simulink model "MATLAB Simulink Model"  (R2020b)
settings: Solver=ode4  StartTime=0.0  StopTime=1  RelTol=1e-3
InitFcn:
  | clear;
  | clc;
  | 
  | %Motor Parameters
  | r1 = 1.405;
  | l1  = 0.005839;
  | r2 = 1.395;
  | l2 = 0.005839;
  | Lm = 0.1722;
  | 
  | %Motor Rated Values
  | Vrat = 400;
  | frat = 50;
  | 
  | x1 = 2*pi*frat*l1;
  | x2 = 2*pi*frat*l2;
  | Xm = 2*pi*frat*Lm;
  | Prat = 4*1000;
  | Nrat = 1430;
  | Ns = 120*frat/4;
  | nrat = Nrat*2*pi/60;
  | ns = Ns*2*pi/60;
  | srat = (Ns-Nrat)/Ns;
  | 
  | E1 = Vrat/sqrt(3); %phase voltage
  | IL = E1/( (r1 + (1i*x1) ) + ( ( (1i*x2) +(r2/srat) )*1i*Xm / ( (1i*Xm) + (1i*x2) + (r2/srat) ) ) );
  | E2 = E1 - (IL*(r1 + (1i*x1) ) );
  | Trat = (3/(ns))*srat*abs(E2)*abs(E2)*r2/((r2*r2) + (srat*srat*x2*x2));
  | %Trat = Prat/nrat;
  | 
  | %System Variables
  | Tsys = (1e-6);
  | Ts = (100e-6);
  | freq = 50;
  | 
  | m=1*freq/50;
  | %m = 1 * (freq/50);
  | Vbus = (400*sqrt(2)*2/sqrt(3)) / (1.15);
  | 
  | Vref = (Vbus*sqrt(3)/2) * m;
  | delay = Ts/Tsys;
  | 
  | % Motor Starting Parameters
  | inc_time = 0.1;
  | 
  | %Motor Loading time
  | load_time = 0.5;
  | 
  | %No. of Hybrid Zones
  | numzones = 3;
  | 
  | %Load ML model Weights
  | 
  | W1R_s1 = readmatrix('Regression Weights\W1_subnet1_tmp_odd_90.xlsx');
  | b1R_s1 = readmatrix('Regression Weights\b1_subnet1_tmp_odd_90.xlsx');
  | W1R_s2 = readmatrix('Regression Weights\W1_subnet2_tmp_odd_90.xlsx');
  | b1R_s2 = readmatrix('Regression Weights\b1_subnet2_tmp_odd_90.xlsx');
  | 
  | W2R = readmatrix('Regression Weights\W2_subnet_tmp_odd_90.xlsx');
  | b2R = readmatrix('Regression Weights\b2_subnet_tmp_odd_90.xlsx');
  | ... (+9 lines)
libraries: powerlib x72, simulink x55, powerlib_meascontrol x15, dspstat3 x11, dspsigops x1
(part 3 of 5)

== system MATLAB Simulink Model/Space Vector PWM based VSI 1/Gating Pulse Generator/Gate Pulse Generator for 2721 Sequence ==
  "S1, S3, S5, sector" : Inport
  AND{,1..5} (6 alike) : Logic  IconShape=distinctive  AllPortsSameDT=off  OutDataTypeStr=boolean
  Constant : Constant  Value=2
  Data Type Conversion : DataTypeConversion
  Demux : Demux
  For Even Sector : Subsystem
  For Odd Sector : Subsystem
  Mod : Math  Operator=mod  SaturateOnIntegerOverflow=on
  Mux : Mux  Inputs=3
  NOT : Logic  Operator=NOT  IconShape=distinctive  AllPortsSameDT=off  OutDataTypeStr=boolean
  OR : Logic  Operator=OR  IconShape=distinctive  AllPortsSameDT=off  OutDataTypeStr=boolean
  OR1 : Logic  Operator=OR  IconShape=distinctive  AllPortsSameDT=off  OutDataTypeStr=boolean
  OR2 : Logic  Operator=OR  IconShape=distinctive  AllPortsSameDT=off  OutDataTypeStr=boolean
  Scope1 : Scope  NumInputPorts=4
  Gate 1 Pulse : Outport
  Gate 3 Pulse : Outport  Port=2
  Gate 5 Pulse : Outport  Port=3
  wires:
  For Even Sector/1(Gate 1 Pulse) -> AND/1
  NOT/1 -> AND2/2, AND1/2, AND/2
  Constant/1 -> Mod/2
  Mux/1 -> For Odd Sector/1("S1, S3, S1"), For Even Sector/1("S1, S3, S5")
  Demux/1 -> Mux/1
  Demux/4 -> Mod/1, Scope1/4
  AND3/1 -> OR/1
  "S1, S3, S5, sector"/1 -> Demux/1
  AND2/1 -> OR2/2
  Data Type Conversion/1 -> NOT/1, AND5/2, AND4/2, AND3/2
  Mod/1 -> Data Type Conversion/1
  AND/1 -> OR/2
  AND1/1 -> OR1/2
  For Odd Sector/2(Gate 3 Pulse) -> AND4/1
  Demux/2 -> Mux/2
  AND5/1 -> OR2/1
  OR/1 -> Gate 1 Pulse/1, Scope1/1
  AND4/1 -> OR1/1
  Demux/3 -> Mux/3
  OR1/1 -> Gate 3 Pulse/1, Scope1/2
  For Even Sector/2(Gate 3 Pulse) -> AND1/1
  OR2/1 -> Gate 5 Pulse/1, Scope1/3
  For Even Sector/3(Gate 5 Pulse) -> AND2/1
  For Odd Sector/1(Gate 1 Pulse) -> AND3/1
  For Odd Sector/3(Gate 5 Pulse) -> AND5/1

== system MATLAB Simulink Model/Space Vector PWM based VSI 1/Gating Pulse Generator/Gate Pulse Generator for 7212 Sequence ==
  "S1, S3, S5, sector" : Inport
  AND{,1..5} (6 alike) : Logic  IconShape=distinctive  AllPortsSameDT=off  OutDataTypeStr=boolean
  Constant : Constant  Value=2
  Data Type Conversion : DataTypeConversion
  Demux : Demux
  For Even Sector : Subsystem
  For Odd Sector : Subsystem
  Mod : Math  Operator=mod  SaturateOnIntegerOverflow=on
  Mux : Mux  Inputs=3
  NOT : Logic  Operator=NOT  IconShape=distinctive  AllPortsSameDT=off  OutDataTypeStr=boolean
  OR : Logic  Operator=OR  IconShape=distinctive  AllPortsSameDT=off  OutDataTypeStr=boolean
  OR1 : Logic  Operator=OR  IconShape=distinctive  AllPortsSameDT=off  OutDataTypeStr=boolean
  OR2 : Logic  Operator=OR  IconShape=distinctive  AllPortsSameDT=off  OutDataTypeStr=boolean
  Scope1 : Scope  NumInputPorts=4
  Gate 1 Pulse : Outport
  Gate 3 Pulse : Outport  Port=2
  Gate 5 Pulse : Outport  Port=3
  wires:
  AND3/1 -> OR/1
  "S1, S3, S5, sector"/1 -> Demux/1
  For Odd Sector/2(Gate 3 Pulse) -> AND4/1
  NOT/1 -> AND2/2, AND1/2, AND/2
  Constant/1 -> Mod/2
  Mux/1 -> For Odd Sector/1("S1, S3, S5"), For Even Sector/1("S1, S3, S1")
  Demux/1 -> Mux/1
  AND2/1 -> OR2/2
  Data Type Conversion/1 -> NOT/1, AND5/2, AND4/2, AND3/2
  Demux/4 -> Mod/1, Scope1/4
  Mod/1 -> Data Type Conversion/1
  AND/1 -> OR/2
  AND1/1 -> OR1/2
  Demux/2 -> Mux/2
  AND5/1 -> OR2/1
  OR/1 -> Gate 1 Pulse/1, Scope1/1
  AND4/1 -> OR1/1
  For Even Sector/1(Gate 1 Pulse) -> AND/1
  Demux/3 -> Mux/3
  OR1/1 -> Gate 3 Pulse/1, Scope1/2
  OR2/1 -> Gate 5 Pulse/1, Scope1/3
  For Even Sector/2(Gate 3 Pulse) -> AND1/1
  For Even Sector/3(Gate 5 Pulse) -> AND2/1
  For Odd Sector/1(Gate 1 Pulse) -> AND3/1
  For Odd Sector/3(Gate 5 Pulse) -> AND5/1

== system MATLAB Simulink Model/Space Vector PWM based VSI 1/Switching Times and Sector/Angle Calculation1 ==
  freq : Inport
  Delay : Delay  DelayLength=1  InitialCondition=0  UseCircularBuffer=on
  Gain1 : Gain  Gain=Tsys
  MATLAB Function : MATLAB Function  TreatAsAtomicUnit=on
  Scope : Scope
  Zero-Order Hold : ZeroOrderHold  SampleTime=Ts
  w : Gain  Gain=2*pi
  wt : Goto  Commented=on  GotoTag=wt  TagVisibility=global
  Angle : Outport
  wires:
  w/1 -> Gain1/1
  MATLAB Function/1(wnew) -> wt/1, Zero-Order Hold/1, Delay/1
  Delay/1 -> MATLAB Function/1(wold)
  Zero-Order Hold/1 -> Angle/1
  Gain1/1 -> MATLAB Function/2(wTs)
  freq/1 -> Scope/1, w/1

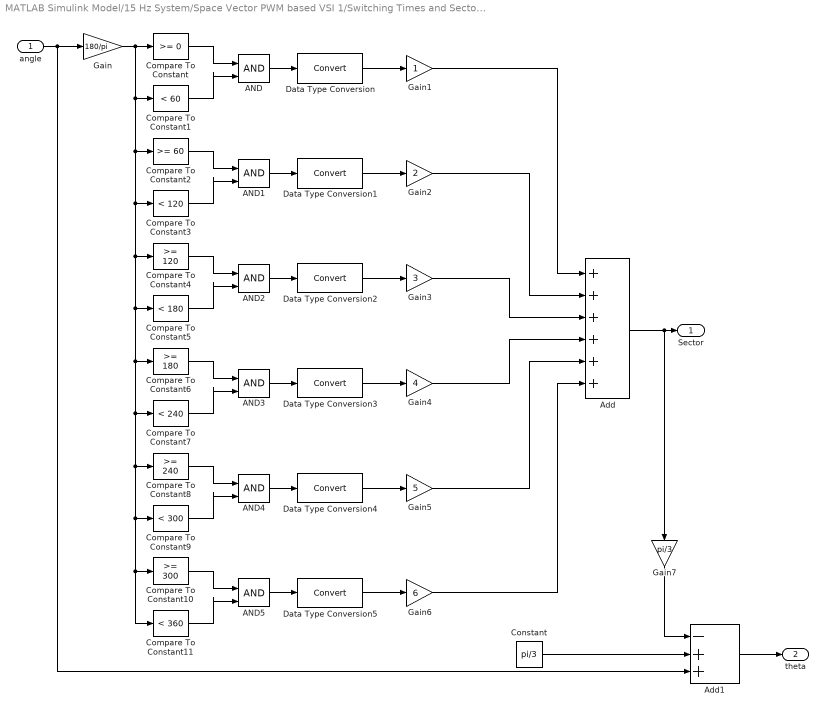
== system MATLAB Simulink Model/15 Hz System/Space Vector PWM based VSI 1/Switching Times and Sector/Angle to Sector and Theta ==
  angle : Inport
  AND{,1..5} (6 alike) : Logic  IconShape=distinctive  AllPortsSameDT=off  OutDataTypeStr=boolean
  Add : Sum  Inputs=++++++
  Add1 : Sum  Inputs=-++
  Compare To Constant : simulink/Logic and Bit Operations/Compare To Constant  relop=>=  const=0  OutDataTypeStr=boolean
  Compare To Constant1 : simulink/Logic and Bit Operations/Compare To Constant  relop=<  const=60  OutDataTypeStr=boolean
  Compare To Constant10 : simulink/Logic and Bit Operations/Compare To Constant  relop=>=  const=300  OutDataTypeStr=boolean
  Compare To Constant11 : simulink/Logic and Bit Operations/Compare To Constant  relop=<  const=360  OutDataTypeStr=boolean
  Compare To Constant2 : simulink/Logic and Bit Operations/Compare To Constant  relop=>=  const=60  OutDataTypeStr=boolean
  Compare To Constant3 : simulink/Logic and Bit Operations/Compare To Constant  relop=<  const=120  OutDataTypeStr=boolean
  Compare To Constant4 : simulink/Logic and Bit Operations/Compare To Constant  relop=>=  const=120  OutDataTypeStr=boolean
  Compare To Constant5 : simulink/Logic and Bit Operations/Compare To Constant  relop=<  const=180  OutDataTypeStr=boolean
  Compare To Constant6 : simulink/Logic and Bit Operations/Compare To Constant  relop=>=  const=180  OutDataTypeStr=boolean
  Compare To Constant7 : simulink/Logic and Bit Operations/Compare To Constant  relop=<  const=240  OutDataTypeStr=boolean
  Compare To Constant8 : simulink/Logic and Bit Operations/Compare To Constant  relop=>=  const=240  OutDataTypeStr=boolean
  Compare To Constant9 : simulink/Logic and Bit Operations/Compare To Constant  relop=<  const=300  OutDataTypeStr=boolean
  Constant : Constant  Value=pi/3
  Data Type Conversion{,1..5} (6 alike) : DataTypeConversion
  Gain : Gain  Gain=180/pi
  Gain1 : Gain
  Gain2 : Gain  Gain=2
  Gain3 : Gain  Gain=3
  Gain4 : Gain  Gain=4
  Gain5 : Gain  Gain=5
  Gain6 : Gain  Gain=6
  Gain7 : Gain  Gain=pi/3
  Sector : Outport
  theta : Outport  Port=2
  wires:
  Add/1 -> Gain7/1, Sector/1
  Gain6/1 -> Add/6
  Gain5/1 -> Add/5
  Gain2/1 -> Add/2
  Gain1/1 -> Add/1
  Gain3/1 -> Add/3
  Gain4/1 -> Add/4
  AND5/1 -> Data Type Conversion5/1
  Data Type Conversion5/1 -> Gain6/1
  Compare To Constant11/1 -> AND5/2
  Compare To Constant10/1 -> AND5/1
  AND4/1 -> Data Type Conversion4/1
  Data Type Conversion4/1 -> Gain5/1
  Compare To Constant9/1 -> AND4/2
  Compare To Constant8/1 -> AND4/1
  AND3/1 -> Data Type Conversion3/1
  Data Type Conversion3/1 -> Gain4/1
  Compare To Constant7/1 -> AND3/2
  Compare To Constant6/1 -> AND3/1
  AND2/1 -> Data Type Conversion2/1
  Data Type Conversion2/1 -> Gain3/1
  Compare To Constant5/1 -> AND2/2
  Compare To Constant4/1 -> AND2/1
  AND1/1 -> Data Type Conversion1/1
  Data Type Conversion1/1 -> Gain2/1
  Compare To Constant3/1 -> AND1/2
  Compare To Constant2/1 -> AND1/1
  Data Type Conversion/1 -> Gain1/1
  AND/1 -> Data Type Conversion/1
  Compare To Constant1/1 -> AND/2
  Compare To Constant/1 -> AND/1
  Gain/1 -> Compare To Constant1/1, Compare To Constant2/1, Compare To Constant3/1, Compare To Constant4/1, Compare To Constant5/1, Compare To Constant6/1, Compare To Constant7/1, Compare To Constant8/1, Compare To Constant9/1, Compare To Constant10/1, Compare To Constant11/1, Compare To Constant/1
  angle/1 -> Add1/3, Gain/1
  Gain7/1 -> Add1/1
  Add1/1 -> theta/1
  Constant/1 -> Add1/2

== system MATLAB Simulink Model/Space Vector PWM based VSI /Gating Pulse Generator/Gate Pulse Generator for 0121 Sequence/For Even Sector ==
  "S1, S3, S5" : Inport
  AND : Logic  IconShape=distinctive  AllPortsSameDT=off  OutDataTypeStr=boolean
  AND1 : Logic  IconShape=distinctive  AllPortsSameDT=off  OutDataTypeStr=boolean
  AND2 : Logic  IconShape=distinctive  AllPortsSameDT=off  OutDataTypeStr=boolean
  Carrier1 : simulink/Sources/Repeating Sequence  rep_seq_t=[0 Ts/2 Ts]  rep_seq_y=[0 Ts-(1e-16) 0]
  Carrier2 : simulink/Sources/Repeating Sequence  rep_seq_t=[0 Ts/2 Ts]  rep_seq_y=[Ts-(1e-16) 0 Ts-(1e-16)]
  Constant : Constant
  Constant1 : Constant  Value=2
  Constant2 : Constant  Value=3
  Demux : Demux  Outputs=3
  GreaterThan{,1..3} (4 alike) : RelationalOperator  OutDataTypeStr=boolean  RndMeth=Simplest
  GreaterThan4 : RelationalOperator  Operator===  OutDataTypeStr=boolean  RndMeth=Simplest
  GreaterThan5 : RelationalOperator  Operator===  OutDataTypeStr=boolean  RndMeth=Simplest
  GreaterThan6 : RelationalOperator  Operator===  OutDataTypeStr=boolean  RndMeth=Simplest
  MATLAB Function : MATLAB Function  TreatAsAtomicUnit=on
  XOR : Logic  Operator=XOR  IconShape=distinctive  AllPortsSameDT=off  OutDataTypeStr=boolean
  XOR1 : Logic  Operator=XOR  IconShape=distinctive  AllPortsSameDT=off  OutDataTypeStr=boolean
  XOR2 : Logic  Operator=XOR  IconShape=distinctive  AllPortsSameDT=off  OutDataTypeStr=boolean
  Gate 1 Pulse : Outport
  Gate 3 Pulse : Outport  Port=2
  Gate 5 Pulse : Outport  Port=3
  wires:
  Demux/3 -> MATLAB Function/3("S5 ")
  Demux/1 -> MATLAB Function/1("S1 ")
  "S1, S3, S5"/1 -> Demux/1
  Demux/2 -> MATLAB Function/2("S3 ")
  MATLAB Function/5(addidx) -> GreaterThan6/2, GreaterThan5/2, GreaterThan4/2
  Constant1/1 -> GreaterThan5/1
  Constant/1 -> GreaterThan4/1
  XOR1/1 -> Gate 3 Pulse/1
  GreaterThan6/1 -> AND2/2
  Constant2/1 -> GreaterThan6/1
  GreaterThan5/1 -> AND1/2
  AND/1 -> XOR/2
  AND2/1 -> XOR2/2
  GreaterThan2/1 -> XOR2/1
  MATLAB Function/1(S1) -> GreaterThan/1
  GreaterThan/1 -> XOR/1
  MATLAB Function/4(addtime) -> GreaterThan3/1
  GreaterThan4/1 -> AND/2
  XOR2/1 -> Gate 5 Pulse/1
  GreaterThan3/1 -> AND/1, AND1/1, AND2/1
  AND1/1 -> XOR1/2
  MATLAB Function/3(S5) -> GreaterThan2/1
  MATLAB Function/2(S3) -> GreaterThan1/1
  XOR/1 -> Gate 1 Pulse/1
  Carrier1/1 -> GreaterThan/2, GreaterThan1/2, GreaterThan2/2
  GreaterThan1/1 -> XOR1/1
  Carrier2/1 -> GreaterThan3/2

== system MATLAB Simulink Model/Space Vector PWM based VSI /Gating Pulse Generator/Gate Pulse Generator for 0121 Sequence/For Odd Sector ==
  "S1, S3, S5" : Inport
  AND : Logic  IconShape=distinctive  AllPortsSameDT=off  OutDataTypeStr=boolean
  AND1 : Logic  IconShape=distinctive  AllPortsSameDT=off  OutDataTypeStr=boolean
  AND2 : Logic  IconShape=distinctive  AllPortsSameDT=off  OutDataTypeStr=boolean
  Carrier1 : simulink/Sources/Repeating Sequence  rep_seq_t=[0 Ts/2 Ts]  rep_seq_y=[Ts-(1e-16) 0 Ts-(1e-16)]
  Constant : Constant
  Constant1 : Constant  Value=2
  Constant2 : Constant  Value=3
  Demux : Demux  Outputs=3
  GreaterThan{,1..3} (4 alike) : RelationalOperator  OutDataTypeStr=boolean  RndMeth=Simplest
  GreaterThan4 : RelationalOperator  Operator===  OutDataTypeStr=boolean  RndMeth=Simplest
  GreaterThan5 : RelationalOperator  Operator===  OutDataTypeStr=boolean  RndMeth=Simplest
  GreaterThan6 : RelationalOperator  Operator===  OutDataTypeStr=boolean  RndMeth=Simplest
  MATLAB Function : MATLAB Function  TreatAsAtomicUnit=on
  XOR : Logic  Operator=XOR  IconShape=distinctive  AllPortsSameDT=off  OutDataTypeStr=boolean
  XOR1 : Logic  Operator=XOR  IconShape=distinctive  AllPortsSameDT=off  OutDataTypeStr=boolean
  XOR2 : Logic  Operator=XOR  IconShape=distinctive  AllPortsSameDT=off  OutDataTypeStr=boolean
  Gate 1 Pulse : Outport
  Gate 3 Pulse : Outport  Port=2
  Gate 5 Pulse : Outport  Port=3
  wires:
  "S1, S3, S5"/1 -> Demux/1
  Demux/1 -> MATLAB Function/1("S1 ")
  Demux/2 -> MATLAB Function/2("S3 ")
  Demux/3 -> MATLAB Function/3("S5 ")
  MATLAB Function/1(S1) -> GreaterThan/1
  Carrier1/1 -> GreaterThan/2, GreaterThan1/2, GreaterThan3/2, GreaterThan2/2
  MATLAB Function/2(S3) -> GreaterThan1/1
  MATLAB Function/3(S5) -> GreaterThan2/1
  MATLAB Function/4(subtime) -> GreaterThan3/1
  MATLAB Function/5(subidx) -> GreaterThan6/2, GreaterThan5/2, GreaterThan4/2
  Constant/1 -> GreaterThan4/1
  Constant1/1 -> GreaterThan5/1
  Constant2/1 -> GreaterThan6/1
  GreaterThan4/1 -> AND/2
  GreaterThan5/1 -> AND1/2
  GreaterThan6/1 -> AND2/2
  GreaterThan3/1 -> AND/1, AND1/1, AND2/1
  AND/1 -> XOR/2
  GreaterThan/1 -> XOR/1
  GreaterThan1/1 -> XOR1/1
  AND1/1 -> XOR1/2
  GreaterThan2/1 -> XOR2/1
  AND2/1 -> XOR2/2
  XOR/1 -> Gate 1 Pulse/1
  XOR1/1 -> Gate 3 Pulse/1
  XOR2/1 -> Gate 5 Pulse/1

== system MATLAB Simulink Model/Space Vector PWM based VSI /Gating Pulse Generator/Gate Pulse Generator for 0127 Sequence 1/For Even Sector ==
  "S1, S3, S5" : Inport
  AND : Logic  IconShape=distinctive  AllPortsSameDT=off  OutDataTypeStr=boolean
  AND1 : Logic  IconShape=distinctive  AllPortsSameDT=off  OutDataTypeStr=boolean
  AND2 : Logic  IconShape=distinctive  AllPortsSameDT=off  OutDataTypeStr=boolean
  Carrier1 : simulink/Sources/Repeating Sequence  rep_seq_t=[0 Ts/2 Ts]  rep_seq_y=[Ts-(1e-16) 0 Ts-(1e-16)]
  Carrier2 : simulink/Sources/Repeating Sequence  rep_seq_t=[0 Ts/2 Ts]  rep_seq_y=[0 Ts-(1e-16) 0]
  Constant : Constant
  Constant1 : Constant  Value=2
  Constant2 : Constant  Value=3
  Demux : Demux  Outputs=3
  GreaterThan{,1..3} (4 alike) : RelationalOperator  OutDataTypeStr=boolean  RndMeth=Simplest
  GreaterThan4 : RelationalOperator  Operator===  OutDataTypeStr=boolean  RndMeth=Simplest
  GreaterThan5 : RelationalOperator  Operator===  OutDataTypeStr=boolean  RndMeth=Simplest
  GreaterThan6 : RelationalOperator  Operator===  OutDataTypeStr=boolean  RndMeth=Simplest
  MATLAB Function : MATLAB Function  TreatAsAtomicUnit=on
  XOR : Logic  Operator=XOR  IconShape=distinctive  AllPortsSameDT=off  OutDataTypeStr=boolean
  XOR1 : Logic  Operator=XOR  IconShape=distinctive  AllPortsSameDT=off  OutDataTypeStr=boolean
  XOR2 : Logic  Operator=XOR  IconShape=distinctive  AllPortsSameDT=off  OutDataTypeStr=boolean
  Gate 1 Pulse : Outport
  Gate 3 Pulse : Outport  Port=2
  Gate 5 Pulse : Outport  Port=3
  wires:
  AND/1 -> XOR/2
  GreaterThan2/1 -> XOR2/1
  "S1, S3, S5"/1 -> Demux/1
  MATLAB Function/1(S1) -> GreaterThan/1
  Demux/1 -> MATLAB Function/1("S1 ")
  Demux/2 -> MATLAB Function/2("S3 ")
  Demux/3 -> MATLAB Function/3("S5 ")
  Carrier2/1 -> GreaterThan3/2
  XOR2/1 -> Gate 5 Pulse/1
  GreaterThan6/1 -> AND2/2
  GreaterThan1/1 -> XOR1/1
  GreaterThan3/1 -> AND/1, AND1/1, AND2/1
  GreaterThan4/1 -> AND/2
  Constant2/1 -> GreaterThan6/1
  AND1/1 -> XOR1/2
  MATLAB Function/2(S3) -> GreaterThan1/1
  MATLAB Function/4(addtime) -> GreaterThan3/1
  XOR/1 -> Gate 1 Pulse/1
  Carrier1/1 -> GreaterThan/2, GreaterThan1/2, GreaterThan2/2
  Constant/1 -> GreaterThan4/1
  MATLAB Function/5(addidx) -> GreaterThan6/2, GreaterThan5/2, GreaterThan4/2
  GreaterThan5/1 -> AND1/2
  GreaterThan/1 -> XOR/1
  XOR1/1 -> Gate 3 Pulse/1
  MATLAB Function/3(S5) -> GreaterThan2/1
  AND2/1 -> XOR2/2
  Constant1/1 -> GreaterThan5/1

== system MATLAB Simulink Model/Space Vector PWM based VSI /Gating Pulse Generator/Gate Pulse Generator for 0127 Sequence 1/For Odd Sector ==
  "S1, S3, S1" : Inport
  AND3 : Logic  IconShape=distinctive  AllPortsSameDT=off  OutDataTypeStr=boolean
  AND4 : Logic  IconShape=distinctive  AllPortsSameDT=off  OutDataTypeStr=boolean
  AND5 : Logic  IconShape=distinctive  AllPortsSameDT=off  OutDataTypeStr=boolean
  Carrier3 : simulink/Sources/Repeating Sequence  rep_seq_t=[0 Ts/2 Ts]  rep_seq_y=[0 Ts-(1e-16) 0]
  Constant3 : Constant
  Constant4 : Constant  Value=2
  Constant5 : Constant  Value=3
  Demux1 : Demux  Outputs=3
  GreaterThan{7..10} (4 alike) : RelationalOperator  OutDataTypeStr=boolean  RndMeth=Simplest
  GreaterThan11 : RelationalOperator  Operator===  OutDataTypeStr=boolean  RndMeth=Simplest
  GreaterThan12 : RelationalOperator  Operator===  OutDataTypeStr=boolean  RndMeth=Simplest
  GreaterThan13 : RelationalOperator  Operator===  OutDataTypeStr=boolean  RndMeth=Simplest
  MATLAB Function1 : MATLAB Function  TreatAsAtomicUnit=on
  XOR3 : Logic  Operator=XOR  IconShape=distinctive  AllPortsSameDT=off  OutDataTypeStr=boolean
  XOR4 : Logic  Operator=XOR  IconShape=distinctive  AllPortsSameDT=off  OutDataTypeStr=boolean
  XOR5 : Logic  Operator=XOR  IconShape=distinctive  AllPortsSameDT=off  OutDataTypeStr=boolean
  Gate 1 Pulse1 : Outport
  Gate 3 Pulse1 : Outport  Port=2
  Gate 5 Pulse1 : Outport  Port=3
  wires:
  GreaterThan12/1 -> AND4/2
  GreaterThan9/1 -> XOR5/1
  Constant4/1 -> GreaterThan12/1
  MATLAB Function1/3(S5) -> GreaterThan9/1
  GreaterThan10/1 -> AND3/1, AND4/1, AND5/1
  MATLAB Function1/5(subidx) -> GreaterThan13/2, GreaterThan12/2, GreaterThan11/2
  MATLAB Function1/2(S3) -> GreaterThan8/1
  AND5/1 -> XOR5/2
  Demux1/2 -> MATLAB Function1/2("S3 ")
  AND4/1 -> XOR4/2
  Demux1/1 -> MATLAB Function1/1("S1 ")
  GreaterThan11/1 -> AND3/2
  AND3/1 -> XOR3/2
  MATLAB Function1/1(S1) -> GreaterThan7/1
  GreaterThan8/1 -> XOR4/1
  GreaterThan13/1 -> AND5/2
  Constant5/1 -> GreaterThan13/1
  GreaterThan7/1 -> XOR3/1
  XOR4/1 -> Gate 3 Pulse1/1
  Demux1/3 -> MATLAB Function1/3("S5 ")
  XOR5/1 -> Gate 5 Pulse1/1
  Constant3/1 -> GreaterThan11/1
  XOR3/1 -> Gate 1 Pulse1/1
  "S1, S3, S1"/1 -> Demux1/1
  Carrier3/1 -> GreaterThan7/2, GreaterThan8/2, GreaterThan10/2, GreaterThan9/2
  MATLAB Function1/4(subtime) -> GreaterThan10/1

== system MATLAB Simulink Model/Space Vector PWM based VSI /Gating Pulse Generator/Gate Pulse Generator for 1012 Sequence/For Even Sector ==
  "S1, S3, S1" : Inport
  AND3 : Logic  IconShape=distinctive  AllPortsSameDT=off  OutDataTypeStr=boolean
  AND4 : Logic  IconShape=distinctive  AllPortsSameDT=off  OutDataTypeStr=boolean
  AND5 : Logic  IconShape=distinctive  AllPortsSameDT=off  OutDataTypeStr=boolean
  Carrier2 : simulink/Sources/Repeating Sequence  rep_seq_t=[0 Ts/2 Ts]  rep_seq_y=[0 Ts-(1e-16) 0]
  Constant3 : Constant
  Constant4 : Constant  Value=2
  Constant5 : Constant  Value=3
  Demux1 : Demux  Outputs=3
  GreaterThan{7..10} (4 alike) : RelationalOperator  OutDataTypeStr=boolean  RndMeth=Simplest
  GreaterThan11 : RelationalOperator  Operator===  OutDataTypeStr=boolean  RndMeth=Simplest
  GreaterThan12 : RelationalOperator  Operator===  OutDataTypeStr=boolean  RndMeth=Simplest
  GreaterThan13 : RelationalOperator  Operator===  OutDataTypeStr=boolean  RndMeth=Simplest
  MATLAB Function1 : MATLAB Function  TreatAsAtomicUnit=on
  XOR3 : Logic  Operator=XOR  IconShape=distinctive  AllPortsSameDT=off  OutDataTypeStr=boolean
  XOR4 : Logic  Operator=XOR  IconShape=distinctive  AllPortsSameDT=off  OutDataTypeStr=boolean
  XOR5 : Logic  Operator=XOR  IconShape=distinctive  AllPortsSameDT=off  OutDataTypeStr=boolean
  Gate 1 Pulse : Outport
  Gate 3 Pulse : Outport  Port=2
  Gate 5 Pulse : Outport  Port=3
  wires:
  XOR3/1 -> Gate 1 Pulse/1
  XOR5/1 -> Gate 5 Pulse/1
  Demux1/3 -> MATLAB Function1/3("S5 ")
  GreaterThan7/1 -> XOR3/1
  GreaterThan11/1 -> AND3/2
  Demux1/2 -> MATLAB Function1/2("S3 ")
  GreaterThan8/1 -> XOR4/1
  XOR4/1 -> Gate 3 Pulse/1
  AND4/1 -> XOR4/2
  AND3/1 -> XOR3/2
  MATLAB Function1/4(subtime) -> GreaterThan10/1
  AND5/1 -> XOR5/2
  GreaterThan13/1 -> AND5/2
  Constant5/1 -> GreaterThan13/1
  Constant3/1 -> GreaterThan11/1
  MATLAB Function1/2(S3) -> GreaterThan8/1
  Demux1/1 -> MATLAB Function1/1("S1 ")
  MATLAB Function1/5(subidx) -> GreaterThan13/2, GreaterThan12/2, GreaterThan11/2
  MATLAB Function1/3(S5) -> GreaterThan9/1
  MATLAB Function1/1(S1) -> GreaterThan7/1
  GreaterThan10/1 -> AND3/1, AND4/1, AND5/1
  Constant4/1 -> GreaterThan12/1
  GreaterThan9/1 -> XOR5/1
  "S1, S3, S1"/1 -> Demux1/1
  Carrier2/1 -> GreaterThan7/2, GreaterThan8/2, GreaterThan10/2, GreaterThan9/2
  GreaterThan12/1 -> AND4/2

== system MATLAB Simulink Model/Space Vector PWM based VSI /Gating Pulse Generator/Gate Pulse Generator for 1012 Sequence/For Odd Sector ==
  "S1, S3, S5" : Inport
  AND : Logic  IconShape=distinctive  AllPortsSameDT=off  OutDataTypeStr=boolean
  AND1 : Logic  IconShape=distinctive  AllPortsSameDT=off  OutDataTypeStr=boolean
  AND2 : Logic  IconShape=distinctive  AllPortsSameDT=off  OutDataTypeStr=boolean
  Carrier1 : simulink/Sources/Repeating Sequence  rep_seq_t=[0 Ts/2 Ts]  rep_seq_y=[Ts-(1e-16) 0 Ts-(1e-16)]
  Carrier2 : simulink/Sources/Repeating Sequence  rep_seq_t=[0 Ts/2 Ts]  rep_seq_y=[0 Ts-(1e-16) 0]
  Constant : Constant
  Constant1 : Constant  Value=2
  Constant2 : Constant  Value=3
  Demux : Demux  Outputs=3
  GreaterThan{,1..3} (4 alike) : RelationalOperator  OutDataTypeStr=boolean  RndMeth=Simplest
  GreaterThan4 : RelationalOperator  Operator===  OutDataTypeStr=boolean  RndMeth=Simplest
  GreaterThan5 : RelationalOperator  Operator===  OutDataTypeStr=boolean  RndMeth=Simplest
  GreaterThan6 : RelationalOperator  Operator===  OutDataTypeStr=boolean  RndMeth=Simplest
  MATLAB Function : MATLAB Function  TreatAsAtomicUnit=on
  XOR : Logic  Operator=XOR  IconShape=distinctive  AllPortsSameDT=off  OutDataTypeStr=boolean
  XOR1 : Logic  Operator=XOR  IconShape=distinctive  AllPortsSameDT=off  OutDataTypeStr=boolean
  XOR2 : Logic  Operator=XOR  IconShape=distinctive  AllPortsSameDT=off  OutDataTypeStr=boolean
  Gate 1 Pulse : Outport
  Gate 3 Pulse : Outport  Port=2
  Gate 5 Pulse : Outport  Port=3
  wires:
  Carrier1/1 -> GreaterThan/2, GreaterThan1/2, GreaterThan2/2
  MATLAB Function/2(S3) -> GreaterThan1/1
  XOR/1 -> Gate 1 Pulse/1
  MATLAB Function/3(S5) -> GreaterThan2/1
  Constant/1 -> GreaterThan4/1
  MATLAB Function/4(addtime) -> GreaterThan3/1
  GreaterThan/1 -> XOR/1
  AND1/1 -> XOR1/2
  GreaterThan3/1 -> AND/1, AND1/1, AND2/1
  GreaterThan1/1 -> XOR1/1
  XOR2/1 -> Gate 5 Pulse/1
  GreaterThan4/1 -> AND/2
  MATLAB Function/1(S1) -> GreaterThan/1
  Carrier2/1 -> GreaterThan3/2
  GreaterThan2/1 -> XOR2/1
  GreaterThan5/1 -> AND1/2
  Constant2/1 -> GreaterThan6/1
  "S1, S3, S5"/1 -> Demux/1
  AND/1 -> XOR/2
  AND2/1 -> XOR2/2
  Constant1/1 -> GreaterThan5/1
  XOR1/1 -> Gate 3 Pulse/1
  MATLAB Function/5(addidx) -> GreaterThan6/2, GreaterThan5/2, GreaterThan4/2
  Demux/3 -> MATLAB Function/3("S5 ")
  Demux/1 -> MATLAB Function/1("S1 ")
  Demux/2 -> MATLAB Function/2("S3 ")
  GreaterThan6/1 -> AND2/2

== system MATLAB Simulink Model/Space Vector PWM based VSI /Gating Pulse Generator/Gate Pulse Generator for 2721 Sequence/For Even Sector ==
  "S1, S3, S5" : Inport
  AND : Logic  IconShape=distinctive  AllPortsSameDT=off  OutDataTypeStr=boolean
  AND1 : Logic  IconShape=distinctive  AllPortsSameDT=off  OutDataTypeStr=boolean
  AND2 : Logic  IconShape=distinctive  AllPortsSameDT=off  OutDataTypeStr=boolean
  Carrier1 : simulink/Sources/Repeating Sequence  rep_seq_t=[0 Ts/2 Ts]  rep_seq_y=[Ts-(1e-16) 0 Ts-(1e-16)]
  Carrier2 : simulink/Sources/Repeating Sequence  rep_seq_t=[0 Ts/2 Ts]  rep_seq_y=[0 Ts-(1e-16) 0]
  Constant : Constant
  Constant1 : Constant  Value=2
  Constant2 : Constant  Value=3
  Demux : Demux  Outputs=3
  GreaterThan{,1..3} (4 alike) : RelationalOperator  OutDataTypeStr=boolean  RndMeth=Simplest
  GreaterThan4 : RelationalOperator  Operator===  OutDataTypeStr=boolean  RndMeth=Simplest
  GreaterThan5 : RelationalOperator  Operator===  OutDataTypeStr=boolean  RndMeth=Simplest
  GreaterThan6 : RelationalOperator  Operator===  OutDataTypeStr=boolean  RndMeth=Simplest
  MATLAB Function : MATLAB Function  TreatAsAtomicUnit=on
  XOR : Logic  Operator=XOR  IconShape=distinctive  AllPortsSameDT=off  OutDataTypeStr=boolean
  XOR1 : Logic  Operator=XOR  IconShape=distinctive  AllPortsSameDT=off  OutDataTypeStr=boolean
  XOR2 : Logic  Operator=XOR  IconShape=distinctive  AllPortsSameDT=off  OutDataTypeStr=boolean
  Gate 1 Pulse : Outport
  Gate 3 Pulse : Outport  Port=2
  Gate 5 Pulse : Outport  Port=3
  wires:
  AND/1 -> XOR/2
  GreaterThan2/1 -> XOR2/1
  "S1, S3, S5"/1 -> Demux/1
  MATLAB Function/1(S1) -> GreaterThan/1
  Demux/1 -> MATLAB Function/1("S1 ")
  Demux/2 -> MATLAB Function/2("S3 ")
  Demux/3 -> MATLAB Function/3("S5 ")
  Carrier2/1 -> GreaterThan3/2
  XOR2/1 -> Gate 5 Pulse/1
  GreaterThan6/1 -> AND2/2
  GreaterThan1/1 -> XOR1/1
  GreaterThan3/1 -> AND/1, AND1/1, AND2/1
  GreaterThan4/1 -> AND/2
  Constant2/1 -> GreaterThan6/1
  AND1/1 -> XOR1/2
  MATLAB Function/2(S3) -> GreaterThan1/1
  MATLAB Function/4(addtime) -> GreaterThan3/1
  XOR/1 -> Gate 1 Pulse/1
  Carrier1/1 -> GreaterThan/2, GreaterThan1/2, GreaterThan2/2
  Constant/1 -> GreaterThan4/1
  MATLAB Function/5(addidx) -> GreaterThan6/2, GreaterThan5/2, GreaterThan4/2
  GreaterThan5/1 -> AND1/2
  GreaterThan/1 -> XOR/1
  XOR1/1 -> Gate 3 Pulse/1
  MATLAB Function/3(S5) -> GreaterThan2/1
  AND2/1 -> XOR2/2
  Constant1/1 -> GreaterThan5/1

== system MATLAB Simulink Model/Space Vector PWM based VSI /Gating Pulse Generator/Gate Pulse Generator for 2721 Sequence/For Odd Sector ==
  "S1, S3, S1" : Inport
  AND3 : Logic  IconShape=distinctive  AllPortsSameDT=off  OutDataTypeStr=boolean
  AND4 : Logic  IconShape=distinctive  AllPortsSameDT=off  OutDataTypeStr=boolean
  AND5 : Logic  IconShape=distinctive  AllPortsSameDT=off  OutDataTypeStr=boolean
  Carrier3 : simulink/Sources/Repeating Sequence  rep_seq_t=[0 Ts/2 Ts]  rep_seq_y=[0 Ts-(1e-16) 0]
  Constant3 : Constant
  Constant4 : Constant  Value=2
  Constant5 : Constant  Value=3
  Demux1 : Demux  Outputs=3
  GreaterThan{7..10} (4 alike) : RelationalOperator  OutDataTypeStr=boolean  RndMeth=Simplest
  GreaterThan11 : RelationalOperator  Operator===  OutDataTypeStr=boolean  RndMeth=Simplest
  GreaterThan12 : RelationalOperator  Operator===  OutDataTypeStr=boolean  RndMeth=Simplest
  GreaterThan13 : RelationalOperator  Operator===  OutDataTypeStr=boolean  RndMeth=Simplest
  MATLAB Function1 : MATLAB Function  TreatAsAtomicUnit=on
  XOR3 : Logic  Operator=XOR  IconShape=distinctive  AllPortsSameDT=off  OutDataTypeStr=boolean
  XOR4 : Logic  Operator=XOR  IconShape=distinctive  AllPortsSameDT=off  OutDataTypeStr=boolean
  XOR5 : Logic  Operator=XOR  IconShape=distinctive  AllPortsSameDT=off  OutDataTypeStr=boolean
  Gate 1 Pulse : Outport
  Gate 3 Pulse : Outport  Port=2
  Gate 5 Pulse : Outport  Port=3
  wires:
  GreaterThan12/1 -> AND4/2
  GreaterThan9/1 -> XOR5/1
  Constant4/1 -> GreaterThan12/1
  MATLAB Function1/3(S5) -> GreaterThan9/1
  GreaterThan10/1 -> AND3/1, AND4/1, AND5/1
  MATLAB Function1/5(subidx) -> GreaterThan13/2, GreaterThan12/2, GreaterThan11/2
  MATLAB Function1/2(S3) -> GreaterThan8/1
  AND5/1 -> XOR5/2
  Demux1/2 -> MATLAB Function1/2("S3 ")
  AND4/1 -> XOR4/2
  Demux1/1 -> MATLAB Function1/1("S1 ")
  GreaterThan11/1 -> AND3/2
  AND3/1 -> XOR3/2
  MATLAB Function1/1(S1) -> GreaterThan7/1
  GreaterThan8/1 -> XOR4/1
  GreaterThan13/1 -> AND5/2
  Constant5/1 -> GreaterThan13/1
  GreaterThan7/1 -> XOR3/1
  XOR4/1 -> Gate 3 Pulse/1
  Demux1/3 -> MATLAB Function1/3("S5 ")
  XOR5/1 -> Gate 5 Pulse/1
  Constant3/1 -> GreaterThan11/1
  XOR3/1 -> Gate 1 Pulse/1
  "S1, S3, S1"/1 -> Demux1/1
  Carrier3/1 -> GreaterThan7/2, GreaterThan8/2, GreaterThan10/2, GreaterThan9/2
  MATLAB Function1/4(subtime) -> GreaterThan10/1

== system MATLAB Simulink Model/Space Vector PWM based VSI /Gating Pulse Generator/Gate Pulse Generator for 7212 Sequence/For Even Sector ==
  "S1, S3, S1" : Inport
  AND3 : Logic  IconShape=distinctive  AllPortsSameDT=off  OutDataTypeStr=boolean
  AND4 : Logic  IconShape=distinctive  AllPortsSameDT=off  OutDataTypeStr=boolean
  AND5 : Logic  IconShape=distinctive  AllPortsSameDT=off  OutDataTypeStr=boolean
  Carrier3 : simulink/Sources/Repeating Sequence  rep_seq_t=[0 Ts/2 Ts]  rep_seq_y=[Ts-(1e-16) 0 Ts-(1e-16)]
  Constant3 : Constant
  Constant4 : Constant  Value=2
  Constant5 : Constant  Value=3
  Demux1 : Demux  Outputs=3
  GreaterThan{7..10} (4 alike) : RelationalOperator  OutDataTypeStr=boolean  RndMeth=Simplest
  GreaterThan11 : RelationalOperator  Operator===  OutDataTypeStr=boolean  RndMeth=Simplest
  GreaterThan12 : RelationalOperator  Operator===  OutDataTypeStr=boolean  RndMeth=Simplest
  GreaterThan13 : RelationalOperator  Operator===  OutDataTypeStr=boolean  RndMeth=Simplest
  MATLAB Function1 : MATLAB Function  TreatAsAtomicUnit=on
  XOR3 : Logic  Operator=XOR  IconShape=distinctive  AllPortsSameDT=off  OutDataTypeStr=boolean
  XOR4 : Logic  Operator=XOR  IconShape=distinctive  AllPortsSameDT=off  OutDataTypeStr=boolean
  XOR5 : Logic  Operator=XOR  IconShape=distinctive  AllPortsSameDT=off  OutDataTypeStr=boolean
  Gate 1 Pulse : Outport
  Gate 3 Pulse : Outport  Port=2
  Gate 5 Pulse : Outport  Port=3
  wires:
  XOR3/1 -> Gate 1 Pulse/1
  XOR5/1 -> Gate 5 Pulse/1
  Demux1/3 -> MATLAB Function1/3("S5 ")
  GreaterThan7/1 -> XOR3/1
  GreaterThan11/1 -> AND3/2
  Demux1/2 -> MATLAB Function1/2("S3 ")
  GreaterThan8/1 -> XOR4/1
  XOR4/1 -> Gate 3 Pulse/1
  AND4/1 -> XOR4/2
  AND3/1 -> XOR3/2
  MATLAB Function1/4(subtime) -> GreaterThan10/1
  AND5/1 -> XOR5/2
  GreaterThan13/1 -> AND5/2
  Constant5/1 -> GreaterThan13/1
  Constant3/1 -> GreaterThan11/1
  MATLAB Function1/2(S3) -> GreaterThan8/1
  Demux1/1 -> MATLAB Function1/1("S1 ")
  MATLAB Function1/5(subidx) -> GreaterThan13/2, GreaterThan12/2, GreaterThan11/2
  MATLAB Function1/3(S5) -> GreaterThan9/1
  MATLAB Function1/1(S1) -> GreaterThan7/1
  GreaterThan10/1 -> AND3/1, AND4/1, AND5/1
  Constant4/1 -> GreaterThan12/1
  GreaterThan9/1 -> XOR5/1
  "S1, S3, S1"/1 -> Demux1/1
  Carrier3/1 -> GreaterThan7/2, GreaterThan8/2, GreaterThan10/2, GreaterThan9/2
  GreaterThan12/1 -> AND4/2

== system MATLAB Simulink Model/Space Vector PWM based VSI /Gating Pulse Generator/Gate Pulse Generator for 7212 Sequence/For Odd Sector ==
  "S1, S3, S5" : Inport
  AND : Logic  IconShape=distinctive  AllPortsSameDT=off  OutDataTypeStr=boolean
  AND1 : Logic  IconShape=distinctive  AllPortsSameDT=off  OutDataTypeStr=boolean
  AND2 : Logic  IconShape=distinctive  AllPortsSameDT=off  OutDataTypeStr=boolean
  Carrier1 : simulink/Sources/Repeating Sequence  rep_seq_t=[0 Ts/2 Ts]  rep_seq_y=[0 Ts-(1e-16) 0]
  Carrier2 : simulink/Sources/Repeating Sequence  rep_seq_t=[0 Ts/2 Ts]  rep_seq_y=[Ts-(1e-16) 0 Ts-(1e-16)]
  Constant : Constant
  Constant1 : Constant  Value=2
  Constant2 : Constant  Value=3
  Demux : Demux  Outputs=3
  GreaterThan{,1..3} (4 alike) : RelationalOperator  OutDataTypeStr=boolean  RndMeth=Simplest
  GreaterThan4 : RelationalOperator  Operator===  OutDataTypeStr=boolean  RndMeth=Simplest
  GreaterThan5 : RelationalOperator  Operator===  OutDataTypeStr=boolean  RndMeth=Simplest
  GreaterThan6 : RelationalOperator  Operator===  OutDataTypeStr=boolean  RndMeth=Simplest
  MATLAB Function : MATLAB Function  TreatAsAtomicUnit=on
  XOR : Logic  Operator=XOR  IconShape=distinctive  AllPortsSameDT=off  OutDataTypeStr=boolean
  XOR1 : Logic  Operator=XOR  IconShape=distinctive  AllPortsSameDT=off  OutDataTypeStr=boolean
  XOR2 : Logic  Operator=XOR  IconShape=distinctive  AllPortsSameDT=off  OutDataTypeStr=boolean
  Gate 1 Pulse : Outport
  Gate 3 Pulse : Outport  Port=2
  Gate 5 Pulse : Outport  Port=3
  wires:
  Carrier1/1 -> GreaterThan/2, GreaterThan1/2, GreaterThan2/2
  MATLAB Function/2(S3) -> GreaterThan1/1
  XOR/1 -> Gate 1 Pulse/1
  MATLAB Function/3(S5) -> GreaterThan2/1
  Constant/1 -> GreaterThan4/1
  MATLAB Function/4(addtime) -> GreaterThan3/1
  GreaterThan/1 -> XOR/1
  AND1/1 -> XOR1/2
  GreaterThan3/1 -> AND/1, AND1/1, AND2/1
  GreaterThan1/1 -> XOR1/1
  XOR2/1 -> Gate 5 Pulse/1
  GreaterThan4/1 -> AND/2
  MATLAB Function/1(S1) -> GreaterThan/1
  Carrier2/1 -> GreaterThan3/2
  GreaterThan2/1 -> XOR2/1
  GreaterThan5/1 -> AND1/2
  Constant2/1 -> GreaterThan6/1
  "S1, S3, S5"/1 -> Demux/1
  AND/1 -> XOR/2
  AND2/1 -> XOR2/2
  Constant1/1 -> GreaterThan5/1
  XOR1/1 -> Gate 3 Pulse/1
  MATLAB Function/5(addidx) -> GreaterThan6/2, GreaterThan5/2, GreaterThan4/2
  Demux/3 -> MATLAB Function/3("S5 ")
  Demux/1 -> MATLAB Function/1("S1 ")
  Demux/2 -> MATLAB Function/2("S3 ")
  GreaterThan6/1 -> AND2/2

== system MATLAB Simulink Model/Space Vector PWM based VSI 1/Gating Pulse Generator/Gate Pulse Generator for 0121 Sequence/For Even Sector ==
  "S1, S3, S5" : Inport
  AND : Logic  IconShape=distinctive  AllPortsSameDT=off  OutDataTypeStr=boolean
  AND1 : Logic  IconShape=distinctive  AllPortsSameDT=off  OutDataTypeStr=boolean
  AND2 : Logic  IconShape=distinctive  AllPortsSameDT=off  OutDataTypeStr=boolean
  Carrier1 : simulink/Sources/Repeating Sequence  rep_seq_t=[0 Ts/2 Ts]  rep_seq_y=[0 Ts-(1e-16) 0]
  Carrier2 : simulink/Sources/Repeating Sequence  rep_seq_t=[0 Ts/2 Ts]  rep_seq_y=[Ts-(1e-16) 0 Ts-(1e-16)]
  Constant : Constant
  Constant1 : Constant  Value=2
  Constant2 : Constant  Value=3
  Demux : Demux  Outputs=3
  GreaterThan{,1..3} (4 alike) : RelationalOperator  OutDataTypeStr=boolean  RndMeth=Simplest
  GreaterThan4 : RelationalOperator  Operator===  OutDataTypeStr=boolean  RndMeth=Simplest
  GreaterThan5 : RelationalOperator  Operator===  OutDataTypeStr=boolean  RndMeth=Simplest
  GreaterThan6 : RelationalOperator  Operator===  OutDataTypeStr=boolean  RndMeth=Simplest
  MATLAB Function : MATLAB Function  TreatAsAtomicUnit=on
  XOR : Logic  Operator=XOR  IconShape=distinctive  AllPortsSameDT=off  OutDataTypeStr=boolean
  XOR1 : Logic  Operator=XOR  IconShape=distinctive  AllPortsSameDT=off  OutDataTypeStr=boolean
  XOR2 : Logic  Operator=XOR  IconShape=distinctive  AllPortsSameDT=off  OutDataTypeStr=boolean
  Gate 1 Pulse : Outport
  Gate 3 Pulse : Outport  Port=2
  Gate 5 Pulse : Outport  Port=3
  wires:
  Carrier2/1 -> GreaterThan3/2
  GreaterThan1/1 -> XOR1/1
  Carrier1/1 -> GreaterThan2/2, GreaterThan1/2, GreaterThan/2
  XOR/1 -> Gate 1 Pulse/1
  MATLAB Function/2(S3) -> GreaterThan1/1
  MATLAB Function/3(S5) -> GreaterThan2/1
  AND1/1 -> XOR1/2
  GreaterThan3/1 -> AND2/1, AND1/1, AND/1
  XOR2/1 -> Gate 5 Pulse/1
  GreaterThan4/1 -> AND/2
  MATLAB Function/4(addtime) -> GreaterThan3/1
  GreaterThan/1 -> XOR/1
  MATLAB Function/1(S1) -> GreaterThan/1
  GreaterThan2/1 -> XOR2/1
  AND2/1 -> XOR2/2
  AND/1 -> XOR/2
  GreaterThan5/1 -> AND1/2
  Constant2/1 -> GreaterThan6/1
  GreaterThan6/1 -> AND2/2
  XOR1/1 -> Gate 3 Pulse/1
  Constant/1 -> GreaterThan4/1
  Constant1/1 -> GreaterThan5/1
  MATLAB Function/5(addidx) -> GreaterThan4/2, GreaterThan5/2, GreaterThan6/2
  Demux/2 -> MATLAB Function/2("S3 ")
  "S1, S3, S5"/1 -> Demux/1
  Demux/1 -> MATLAB Function/1("S1 ")
  Demux/3 -> MATLAB Function/3("S5 ")

== system MATLAB Simulink Model/Space Vector PWM based VSI 1/Gating Pulse Generator/Gate Pulse Generator for 0121 Sequence/For Odd Sector ==
  "S1, S3, S5" : Inport
  AND : Logic  IconShape=distinctive  AllPortsSameDT=off  OutDataTypeStr=boolean
  AND1 : Logic  IconShape=distinctive  AllPortsSameDT=off  OutDataTypeStr=boolean
  AND2 : Logic  IconShape=distinctive  AllPortsSameDT=off  OutDataTypeStr=boolean
  Carrier1 : simulink/Sources/Repeating Sequence  rep_seq_t=[0 Ts/2 Ts]  rep_seq_y=[Ts-(1e-16) 0 Ts-(1e-16)]
  Constant : Constant
  Constant1 : Constant  Value=2
  Constant2 : Constant  Value=3
  Demux : Demux  Outputs=3
  GreaterThan{,1..3} (4 alike) : RelationalOperator  OutDataTypeStr=boolean  RndMeth=Simplest
  GreaterThan4 : RelationalOperator  Operator===  OutDataTypeStr=boolean  RndMeth=Simplest
  GreaterThan5 : RelationalOperator  Operator===  OutDataTypeStr=boolean  RndMeth=Simplest
  GreaterThan6 : RelationalOperator  Operator===  OutDataTypeStr=boolean  RndMeth=Simplest
  MATLAB Function : MATLAB Function  TreatAsAtomicUnit=on
  XOR : Logic  Operator=XOR  IconShape=distinctive  AllPortsSameDT=off  OutDataTypeStr=boolean
  XOR1 : Logic  Operator=XOR  IconShape=distinctive  AllPortsSameDT=off  OutDataTypeStr=boolean
  XOR2 : Logic  Operator=XOR  IconShape=distinctive  AllPortsSameDT=off  OutDataTypeStr=boolean
  Gate 1 Pulse : Outport
  Gate 3 Pulse : Outport  Port=2
  Gate 5 Pulse : Outport  Port=3
  wires:
  XOR2/1 -> Gate 5 Pulse/1
  XOR1/1 -> Gate 3 Pulse/1
  XOR/1 -> Gate 1 Pulse/1
  AND2/1 -> XOR2/2
  GreaterThan2/1 -> XOR2/1
  AND1/1 -> XOR1/2
  GreaterThan1/1 -> XOR1/1
  GreaterThan/1 -> XOR/1
  AND/1 -> XOR/2
  GreaterThan3/1 -> AND2/1, AND1/1, AND/1
  GreaterThan6/1 -> AND2/2
  GreaterThan5/1 -> AND1/2
  GreaterThan4/1 -> AND/2
  Constant2/1 -> GreaterThan6/1
  Constant1/1 -> GreaterThan5/1
  Constant/1 -> GreaterThan4/1
  MATLAB Function/5(subidx) -> GreaterThan4/2, GreaterThan5/2, GreaterThan6/2
  MATLAB Function/4(subtime) -> GreaterThan3/1
  MATLAB Function/3(S5) -> GreaterThan2/1
  MATLAB Function/2(S3) -> GreaterThan1/1
  Carrier1/1 -> GreaterThan2/2, GreaterThan3/2, GreaterThan1/2, GreaterThan/2
  MATLAB Function/1(S1) -> GreaterThan/1
  Demux/3 -> MATLAB Function/3("S5 ")
  Demux/2 -> MATLAB Function/2("S3 ")
  Demux/1 -> MATLAB Function/1("S1 ")
  "S1, S3, S5"/1 -> Demux/1

== system MATLAB Simulink Model/Space Vector PWM based VSI 1/Gating Pulse Generator/Gate Pulse Generator for 0127 Sequence 1/For Even Sector ==
  "S1, S3, S5" : Inport
  AND : Logic  IconShape=distinctive  AllPortsSameDT=off  OutDataTypeStr=boolean
  AND1 : Logic  IconShape=distinctive  AllPortsSameDT=off  OutDataTypeStr=boolean
  AND2 : Logic  IconShape=distinctive  AllPortsSameDT=off  OutDataTypeStr=boolean
  Carrier1 : simulink/Sources/Repeating Sequence  rep_seq_t=[0 Ts/2 Ts]  rep_seq_y=[Ts-(1e-16) 0 Ts-(1e-16)]
  Carrier2 : simulink/Sources/Repeating Sequence  rep_seq_t=[0 Ts/2 Ts]  rep_seq_y=[0 Ts-(1e-16) 0]
  Constant : Constant
  Constant1 : Constant  Value=2
  Constant2 : Constant  Value=3
  Demux : Demux  Outputs=3
  GreaterThan{,1..3} (4 alike) : RelationalOperator  OutDataTypeStr=boolean  RndMeth=Simplest
  GreaterThan4 : RelationalOperator  Operator===  OutDataTypeStr=boolean  RndMeth=Simplest
  GreaterThan5 : RelationalOperator  Operator===  OutDataTypeStr=boolean  RndMeth=Simplest
  GreaterThan6 : RelationalOperator  Operator===  OutDataTypeStr=boolean  RndMeth=Simplest
  MATLAB Function : MATLAB Function  TreatAsAtomicUnit=on
  XOR : Logic  Operator=XOR  IconShape=distinctive  AllPortsSameDT=off  OutDataTypeStr=boolean
  XOR1 : Logic  Operator=XOR  IconShape=distinctive  AllPortsSameDT=off  OutDataTypeStr=boolean
  XOR2 : Logic  Operator=XOR  IconShape=distinctive  AllPortsSameDT=off  OutDataTypeStr=boolean
  Gate 1 Pulse : Outport
  Gate 3 Pulse : Outport  Port=2
  Gate 5 Pulse : Outport  Port=3
  wires:
  Constant1/1 -> GreaterThan5/1
  AND2/1 -> XOR2/2
  MATLAB Function/3(S5) -> GreaterThan2/1
  XOR1/1 -> Gate 3 Pulse/1
  GreaterThan/1 -> XOR/1
  GreaterThan5/1 -> AND1/2
  MATLAB Function/5(addidx) -> GreaterThan4/2, GreaterThan5/2, GreaterThan6/2
  Constant/1 -> GreaterThan4/1
  Carrier1/1 -> GreaterThan2/2, GreaterThan1/2, GreaterThan/2
  XOR/1 -> Gate 1 Pulse/1
  MATLAB Function/4(addtime) -> GreaterThan3/1
  MATLAB Function/2(S3) -> GreaterThan1/1
  AND1/1 -> XOR1/2
  Constant2/1 -> GreaterThan6/1
  GreaterThan4/1 -> AND/2
  GreaterThan3/1 -> AND2/1, AND1/1, AND/1
  GreaterThan1/1 -> XOR1/1
  GreaterThan6/1 -> AND2/2
  XOR2/1 -> Gate 5 Pulse/1
  Carrier2/1 -> GreaterThan3/2
  Demux/3 -> MATLAB Function/3("S5 ")
  Demux/2 -> MATLAB Function/2("S3 ")
  Demux/1 -> MATLAB Function/1("S1 ")
  MATLAB Function/1(S1) -> GreaterThan/1
  "S1, S3, S5"/1 -> Demux/1
  GreaterThan2/1 -> XOR2/1
  AND/1 -> XOR/2

== system MATLAB Simulink Model/Space Vector PWM based VSI 1/Gating Pulse Generator/Gate Pulse Generator for 0127 Sequence 1/For Odd Sector ==
  "S1, S3, S1" : Inport
  AND3 : Logic  IconShape=distinctive  AllPortsSameDT=off  OutDataTypeStr=boolean
  AND4 : Logic  IconShape=distinctive  AllPortsSameDT=off  OutDataTypeStr=boolean
  AND5 : Logic  IconShape=distinctive  AllPortsSameDT=off  OutDataTypeStr=boolean
  Carrier3 : simulink/Sources/Repeating Sequence  rep_seq_t=[0 Ts/2 Ts]  rep_seq_y=[0 Ts-(1e-16) 0]
  Constant3 : Constant
  Constant4 : Constant  Value=2
  Constant5 : Constant  Value=3
  Demux1 : Demux  Outputs=3
  GreaterThan{7..10} (4 alike) : RelationalOperator  OutDataTypeStr=boolean  RndMeth=Simplest
  GreaterThan11 : RelationalOperator  Operator===  OutDataTypeStr=boolean  RndMeth=Simplest
  GreaterThan12 : RelationalOperator  Operator===  OutDataTypeStr=boolean  RndMeth=Simplest
  GreaterThan13 : RelationalOperator  Operator===  OutDataTypeStr=boolean  RndMeth=Simplest
  MATLAB Function1 : MATLAB Function  TreatAsAtomicUnit=on
  XOR3 : Logic  Operator=XOR  IconShape=distinctive  AllPortsSameDT=off  OutDataTypeStr=boolean
  XOR4 : Logic  Operator=XOR  IconShape=distinctive  AllPortsSameDT=off  OutDataTypeStr=boolean
  XOR5 : Logic  Operator=XOR  IconShape=distinctive  AllPortsSameDT=off  OutDataTypeStr=boolean
  Gate 1 Pulse1 : Outport
  Gate 3 Pulse1 : Outport  Port=2
  Gate 5 Pulse1 : Outport  Port=3
  wires:
  MATLAB Function1/4(subtime) -> GreaterThan10/1
  Carrier3/1 -> GreaterThan9/2, GreaterThan10/2, GreaterThan8/2, GreaterThan7/2
  "S1, S3, S1"/1 -> Demux1/1
  XOR3/1 -> Gate 1 Pulse1/1
  Constant3/1 -> GreaterThan11/1
  XOR5/1 -> Gate 5 Pulse1/1
  Demux1/3 -> MATLAB Function1/3("S5 ")
  XOR4/1 -> Gate 3 Pulse1/1
  GreaterThan7/1 -> XOR3/1
  Constant5/1 -> GreaterThan13/1
  GreaterThan13/1 -> AND5/2
  GreaterThan8/1 -> XOR4/1
  MATLAB Function1/1(S1) -> GreaterThan7/1
  AND3/1 -> XOR3/2
  GreaterThan11/1 -> AND3/2
  Demux1/1 -> MATLAB Function1/1("S1 ")
  AND4/1 -> XOR4/2
  Demux1/2 -> MATLAB Function1/2("S3 ")
  AND5/1 -> XOR5/2
  MATLAB Function1/2(S3) -> GreaterThan8/1
  MATLAB Function1/5(subidx) -> GreaterThan11/2, GreaterThan12/2, GreaterThan13/2
  GreaterThan10/1 -> AND5/1, AND4/1, AND3/1
  MATLAB Function1/3(S5) -> GreaterThan9/1
  Constant4/1 -> GreaterThan12/1
  GreaterThan9/1 -> XOR5/1
  GreaterThan12/1 -> AND4/2

== system MATLAB Simulink Model/Space Vector PWM based VSI 1/Gating Pulse Generator/Gate Pulse Generator for 1012 Sequence/For Even Sector ==
  "S1, S3, S1" : Inport
  AND3 : Logic  IconShape=distinctive  AllPortsSameDT=off  OutDataTypeStr=boolean
  AND4 : Logic  IconShape=distinctive  AllPortsSameDT=off  OutDataTypeStr=boolean
  AND5 : Logic  IconShape=distinctive  AllPortsSameDT=off  OutDataTypeStr=boolean
  Carrier2 : simulink/Sources/Repeating Sequence  rep_seq_t=[0 Ts/2 Ts]  rep_seq_y=[0 Ts-(1e-16) 0]
  Constant3 : Constant
  Constant4 : Constant  Value=2
  Constant5 : Constant  Value=3
  Demux1 : Demux  Outputs=3
  GreaterThan{7..10} (4 alike) : RelationalOperator  OutDataTypeStr=boolean  RndMeth=Simplest
  GreaterThan11 : RelationalOperator  Operator===  OutDataTypeStr=boolean  RndMeth=Simplest
  GreaterThan12 : RelationalOperator  Operator===  OutDataTypeStr=boolean  RndMeth=Simplest
  GreaterThan13 : RelationalOperator  Operator===  OutDataTypeStr=boolean  RndMeth=Simplest
  MATLAB Function1 : MATLAB Function  TreatAsAtomicUnit=on
  XOR3 : Logic  Operator=XOR  IconShape=distinctive  AllPortsSameDT=off  OutDataTypeStr=boolean
  XOR4 : Logic  Operator=XOR  IconShape=distinctive  AllPortsSameDT=off  OutDataTypeStr=boolean
  XOR5 : Logic  Operator=XOR  IconShape=distinctive  AllPortsSameDT=off  OutDataTypeStr=boolean
  Gate 1 Pulse : Outport
  Gate 3 Pulse : Outport  Port=2
  Gate 5 Pulse : Outport  Port=3
  wires:
  GreaterThan12/1 -> AND4/2
  Carrier2/1 -> GreaterThan9/2, GreaterThan10/2, GreaterThan8/2, GreaterThan7/2
  "S1, S3, S1"/1 -> Demux1/1
  GreaterThan9/1 -> XOR5/1
  Constant4/1 -> GreaterThan12/1
  GreaterThan10/1 -> AND5/1, AND4/1, AND3/1
  MATLAB Function1/1(S1) -> GreaterThan7/1
  MATLAB Function1/3(S5) -> GreaterThan9/1
  MATLAB Function1/5(subidx) -> GreaterThan11/2, GreaterThan12/2, GreaterThan13/2
  Demux1/1 -> MATLAB Function1/1("S1 ")
  MATLAB Function1/2(S3) -> GreaterThan8/1
  Constant3/1 -> GreaterThan11/1
  Constant5/1 -> GreaterThan13/1
  GreaterThan13/1 -> AND5/2
  AND5/1 -> XOR5/2
  MATLAB Function1/4(subtime) -> GreaterThan10/1
  AND3/1 -> XOR3/2
  AND4/1 -> XOR4/2
  XOR4/1 -> Gate 3 Pulse/1
  GreaterThan8/1 -> XOR4/1
  Demux1/2 -> MATLAB Function1/2("S3 ")
  GreaterThan11/1 -> AND3/2
  GreaterThan7/1 -> XOR3/1
  Demux1/3 -> MATLAB Function1/3("S5 ")
  XOR5/1 -> Gate 5 Pulse/1
  XOR3/1 -> Gate 1 Pulse/1

== system MATLAB Simulink Model/Space Vector PWM based VSI 1/Gating Pulse Generator/Gate Pulse Generator for 1012 Sequence/For Odd Sector ==
  "S1, S3, S5" : Inport
  AND : Logic  IconShape=distinctive  AllPortsSameDT=off  OutDataTypeStr=boolean
  AND1 : Logic  IconShape=distinctive  AllPortsSameDT=off  OutDataTypeStr=boolean
  AND2 : Logic  IconShape=distinctive  AllPortsSameDT=off  OutDataTypeStr=boolean
  Carrier1 : simulink/Sources/Repeating Sequence  rep_seq_t=[0 Ts/2 Ts]  rep_seq_y=[Ts-(1e-16) 0 Ts-(1e-16)]
  Carrier2 : simulink/Sources/Repeating Sequence  rep_seq_t=[0 Ts/2 Ts]  rep_seq_y=[0 Ts-(1e-16) 0]
  Constant : Constant
  Constant1 : Constant  Value=2
  Constant2 : Constant  Value=3
  Demux : Demux  Outputs=3
  GreaterThan{,1..3} (4 alike) : RelationalOperator  OutDataTypeStr=boolean  RndMeth=Simplest
  GreaterThan4 : RelationalOperator  Operator===  OutDataTypeStr=boolean  RndMeth=Simplest
  GreaterThan5 : RelationalOperator  Operator===  OutDataTypeStr=boolean  RndMeth=Simplest
  GreaterThan6 : RelationalOperator  Operator===  OutDataTypeStr=boolean  RndMeth=Simplest
  MATLAB Function : MATLAB Function  TreatAsAtomicUnit=on
  XOR : Logic  Operator=XOR  IconShape=distinctive  AllPortsSameDT=off  OutDataTypeStr=boolean
  XOR1 : Logic  Operator=XOR  IconShape=distinctive  AllPortsSameDT=off  OutDataTypeStr=boolean
  XOR2 : Logic  Operator=XOR  IconShape=distinctive  AllPortsSameDT=off  OutDataTypeStr=boolean
  Gate 1 Pulse : Outport
  Gate 3 Pulse : Outport  Port=2
  Gate 5 Pulse : Outport  Port=3
  wires:
  GreaterThan6/1 -> AND2/2
  Demux/2 -> MATLAB Function/2("S3 ")
  Demux/1 -> MATLAB Function/1("S1 ")
  Demux/3 -> MATLAB Function/3("S5 ")
  MATLAB Function/5(addidx) -> GreaterThan4/2, GreaterThan5/2, GreaterThan6/2
  XOR1/1 -> Gate 3 Pulse/1
  Constant1/1 -> GreaterThan5/1
  AND2/1 -> XOR2/2
  AND/1 -> XOR/2
  "S1, S3, S5"/1 -> Demux/1
  Constant2/1 -> GreaterThan6/1
  GreaterThan5/1 -> AND1/2
  GreaterThan2/1 -> XOR2/1
  Carrier2/1 -> GreaterThan3/2
  MATLAB Function/1(S1) -> GreaterThan/1
  GreaterThan4/1 -> AND/2
  XOR2/1 -> Gate 5 Pulse/1
  GreaterThan1/1 -> XOR1/1
  GreaterThan3/1 -> AND2/1, AND1/1, AND/1
  AND1/1 -> XOR1/2
  GreaterThan/1 -> XOR/1
  MATLAB Function/4(addtime) -> GreaterThan3/1
  Constant/1 -> GreaterThan4/1
  MATLAB Function/3(S5) -> GreaterThan2/1
  XOR/1 -> Gate 1 Pulse/1
  MATLAB Function/2(S3) -> GreaterThan1/1
  Carrier1/1 -> GreaterThan2/2, GreaterThan1/2, GreaterThan/2
